simulink model "ur5_simulink_control_2023b"  (R2023b)
settings: Solver=FixedStepAuto  StartTime=0.0  StopTime=inf  FixedStep=0.04  RelTol=1e-3
undefined symbols (not defined in the file or in its folder): data
libraries: robotmaniplib x14, robotcorelib x7, vrlib x2, eeGeneralControl x1
settings Model: Creator=81232  LastModifiedBy=ASUS

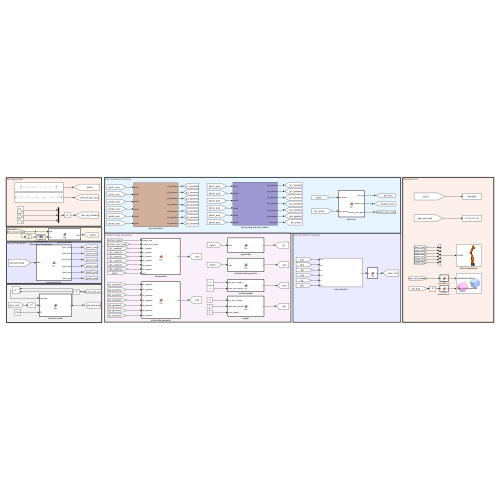
[thumbnail: Simulink's stored preview of the top-level diagram]
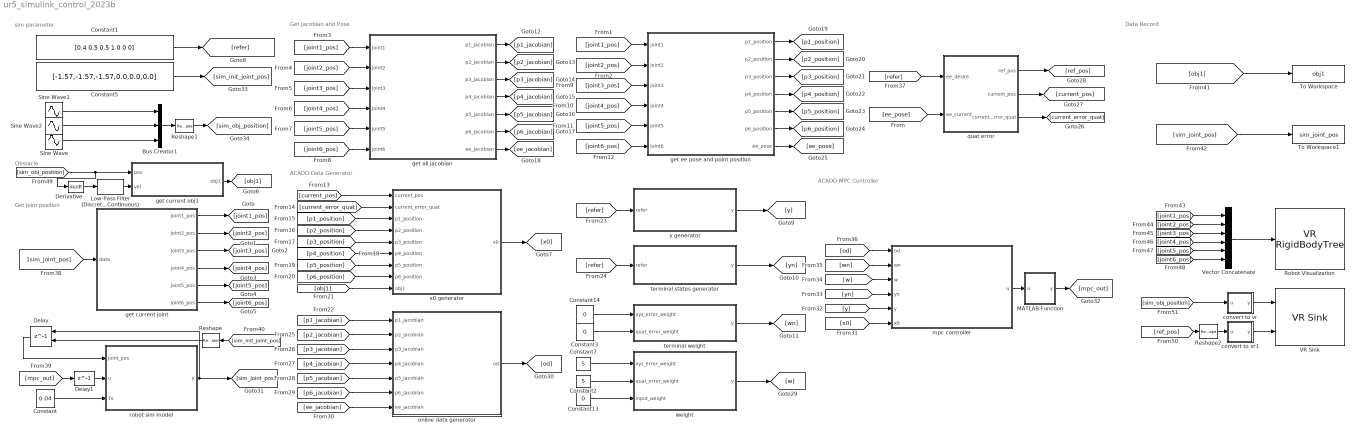
== system ur5_simulink_control_2023b ==
  note: sim parameter
  note: Get joint position
  note: Data Record
  note: Obstacle
  note: ACADO MPC Controller
  note: Get Jacobian and Pose
  note: ACADO Data Generator
  Bus Creator1 : BusCreator  Inputs=3
  Constant : Constant  Value=0.04
  Constant1 : Constant  Value=[0.4 0.5 0.5 1 0 0 0]
  Constant13 : Constant  Value=0
  Constant14 : Constant  Value=0
  Constant2 : Constant  Value=5
  Constant3 : Constant  Value=0
  Constant5 : Constant  Value=[-1.57,-1.57,-1.57,0.0,0.0,0.0]  VectorParams1D=off
  Constant7 : Constant  Value=5
  Delay : Delay  DelayLength=1  InitialConditionSource=Input port  InitialCondition=1
      settings: InputPortMap=u0,p4
  Delay1 : Delay  DelayLength=1
  Derivative : Derivative
  Low-Pass Filter (Discrete or Continuous) : eeGeneralControl/Low-Pass Filter (Discrete or Continuous)  K=1  T=1  B=inf  A=-inf  init_option=Inherited from block input  x0=0  Ts=-1
  MATLAB Function : MATLAB Function  TreatAsAtomicUnit=on
  Reshape : Reshape  OutputDimensionality=Customize  OutputDimensions=[1,6]
  Reshape1 : Reshape  OutputDimensionality=Customize  OutputDimensions=[1,3]
  Reshape2 : Reshape  OutputDimensionality=Customize  OutputDimensions=[1,3]
  Robot Visualization : vrlib/VR RigidBodyTree  VrmlFile=obstacle_robot_scene.x3d  RBT=ur5_model  useRBT=off  Ts=-1  ForceViewerOpen=on
  Sine Wave : Sin  Amplitude=0.3  Bias=0.4  Frequency=0.8  SampleTime=0
  Sine Wave1 : Sin  Amplitude=0.3  Bias=0.4  Frequency=0  SampleTime=0
  Sine Wave2 : Sin  Amplitude=0.3  Bias=0.5  Frequency=0.8  SampleTime=0
  To Workspace : ToWorkspace  VariableName=obj1  SaveFormat=Timeseries  SampleTime=-1
  To Workspace1 : ToWorkspace  VariableName=sim_joint_pos  SaveFormat=Timeseries  SampleTime=-1
  VR Sink : vrlib/VR Sink  InstantiateOnLoad=on  SampleTime=-1  ViewEnable=on  RemoteChange=off  RemoteView=off  FieldsWritten=obstacle.translation.3.1.1.double#refer_point.translation.3.1.1.double  WorldFileName=obstacle_robot_scene.x3d  WorldDescription=Simple Robot Scene  AutoView=off  VideoDimensions=[]  AllowVariableSize=off  FigureProperties=[]
  Vector Concatenate : Concatenate  NumInputs=6
  convert to vr : MATLAB Function  TreatAsAtomicUnit=on
  convert to vr1 : MATLAB Function  TreatAsAtomicUnit=on
  get all jacobian : Subsystem
  get current joint : MATLAB Function  TreatAsAtomicUnit=on
  get current obj1 : MATLAB Function  TreatAsAtomicUnit=on
  get ee pose and point position : Subsystem
  mpc controller : Subsystem
  online data generator : MATLAB Function  TreatAsAtomicUnit=on
  quat error : MATLAB Function  TreatAsAtomicUnit=on
  robot sim model : MATLAB Function  TreatAsAtomicUnit=on
  terminal states generator : MATLAB Function  TreatAsAtomicUnit=on
  terminal weight : MATLAB Function  TreatAsAtomicUnit=on
  weight : MATLAB Function  TreatAsAtomicUnit=on
  x0 generator : MATLAB Function  TreatAsAtomicUnit=on
  y generator : MATLAB Function  TreatAsAtomicUnit=on
  wires:
  get current joint/1(joint1_pos) -> [joint1_pos]
  get current joint/2(joint2_pos) -> [joint2_pos]
  get current joint/3(joint3_pos) -> [joint3_pos]
  get current joint/4(joint4_pos) -> [joint4_pos]
  get current joint/5(joint5_pos) -> [joint5_pos]
  get current joint/6(joint6_pos) -> [joint6_pos]
  [joint1_pos] -> get all jacobian/1(joint1)
  [joint2_pos] -> get all jacobian/2(joint2)
  [joint3_pos] -> get all jacobian/3(joint3)
  [joint4_pos] -> get all jacobian/4(joint4)
  [joint5_pos] -> get all jacobian/5(joint5)
  [joint6_pos] -> get all jacobian/6(joint6)
  get all jacobian/1(p1_jacobian) -> [p1_jacobian]
  get all jacobian/2(p2_jacobian) -> [p2_jacobian]
  get all jacobian/3(p3_jacobian) -> [p3_jacobian]
  get all jacobian/4(p4_jacobian) -> [p4_jacobian]
  get all jacobian/5(p5_jacobian) -> [p5_jacobian]
  get all jacobian/6(p6_jacobian) -> [p6_jacobian]
  get all jacobian/7(ee_jacobian) -> [ee_jacobian]
  [joint6_pos] -> get ee pose and point position/6(joint6)
  [joint4_pos] -> get ee pose and point position/4(joint4)
  [joint1_pos] -> get ee pose and point position/1(joint1)
  [joint2_pos] -> get ee pose and point position/2(joint2)
  [joint5_pos] -> get ee pose and point position/5(joint5)
  [joint3_pos] -> get ee pose and point position/3(joint3)
  [refer] -> quat error/1(ee_desire)
  quat error/3(current_error_quat) -> [current_error_quat]
  get current obj1/1(obj1) -> [obj1]
  get ee pose and point position/1(p1_position) -> [p1_position]
  get ee pose and point position/2(p2_position) -> [p2_position]
  get ee pose and point position/3(p3_position) -> [p3_position]
  get ee pose and point position/4(p4_position) -> [p4_position]
  get ee pose and point position/5(p5_position) -> [p5_position]
  get ee pose and point position/6(p6_position) -> [p6_position]
  get ee pose and point position/7(ee_pose) -> [ee_pose]
  [ee_pose] -> quat error/2(ee_current)
  quat error/2(current_pos) -> [current_pos]
  quat error/1(ref_pos) -> [ref_pos]
  [current_pos] -> x0 generator/1(current_pos)
  [current_error_quat] -> x0 generator/2(current_error_quat)
  [p1_position] -> x0 generator/3(p1_position)
  [p2_position] -> x0 generator/4(p2_position)
  [p3_position] -> x0 generator/5(p3_position)
  [p4_position] -> x0 generator/6(p4_position)
  [p5_position] -> x0 generator/7(p5_position)
  [p6_position] -> x0 generator/8(p6_position)
  [obj1] -> x0 generator/9(obj1)
  x0 generator/1(x0) -> [x0]
  Constant1/1 -> [refer]
  [refer] -> terminal states generator/1(refer)
  terminal states generator/1(y) -> [yn]
  y generator/1(y) -> [y]
  [refer] -> y generator/1(refer)
  terminal weight/1(y) -> [wn]
  Constant7/1 -> weight/1(xyz_error_weight)
  weight/1(y) -> [w]
  Constant14/1 -> terminal weight/1(xyz_error_weight)
  Constant13/1 -> weight/3(input_weight)
  Constant2/1 -> weight/2(quat_error_weight)
  Constant3/1 -> terminal weight/2(quat_error_weight)
  [p1_jacobian] -> online data generator/1(p1_jacobian)
  [p2_jacobian] -> online data generator/2(p2_jacobian)
  [p3_jacobian] -> online data generator/3(p3_jacobian)
  [p4_jacobian] -> online data generator/4(p4_jacobian)
  [p5_jacobian] -> online data generator/5(p5_jacobian)
  [p6_jacobian] -> online data generator/6(p6_jacobian)
  [ee_jacobian] -> online data generator/7(ee_jacobian)
  online data generator/1(od) -> [od]
  [od] -> mpc controller/1(od)
  [wn] -> mpc controller/2(wn)
  [w] -> mpc controller/3(w)
  [yn] -> mpc controller/4(yn)
  [y] -> mpc controller/5(y)
  [x0] -> mpc controller/6(x0)
  Constant/1 -> robot sim model/3(Ts)
  robot sim model/1(y) -> [sim_joint_pos], Delay/1
  Delay/1 -> robot sim model/1(joint_pos)
  [sim_init_joint_pos] -> Reshape/1
  [sim_joint_pos] -> get current joint/1(data)
  Delay1/1 -> robot sim model/2(u)
  Reshape/1 -> Delay/2
  mpc controller/1(u) -> MATLAB Function/1(u)
  MATLAB Function/1(y) -> [mpc_out]
  Constant5/1 -> [sim_init_joint_pos]
  [mpc_out] -> Delay1/1
  [obj1] -> To Workspace/1
  [sim_joint_pos] -> To Workspace1/1
  Vector Concatenate/1 -> Robot Visualization/1
  [joint3_pos] -> Vector Concatenate/3
  [joint1_pos] -> Vector Concatenate/1
  [joint2_pos] -> Vector Concatenate/2
  [joint5_pos] -> Vector Concatenate/5
  [joint6_pos] -> Vector Concatenate/6
  [joint4_pos] -> Vector Concatenate/4
  Reshape1/1 -> [sim_obj_position]
  [sim_obj_position] -> Derivative/1, get current obj1/1(pos)
  [sim_obj_position] -> convert to vr/1(u)
  Sine Wave2/1 -> Bus Creator1/2
  Bus Creator1/1 -> Reshape1/1
  Sine Wave1/1 -> Bus Creator1/1
  Sine Wave/1 -> Bus Creator1/3
  Derivative/1 -> Low-Pass Filter (Discrete or Continuous)/1
  Low-Pass Filter (Discrete or Continuous)/1 -> get current obj1/2(vel)
  convert to vr/1(y) -> VR Sink/1
  convert to vr1/1(y) -> VR Sink/2
  Reshape2/1 -> convert to vr1/1(u)
  [ref_pos] -> Reshape2/1

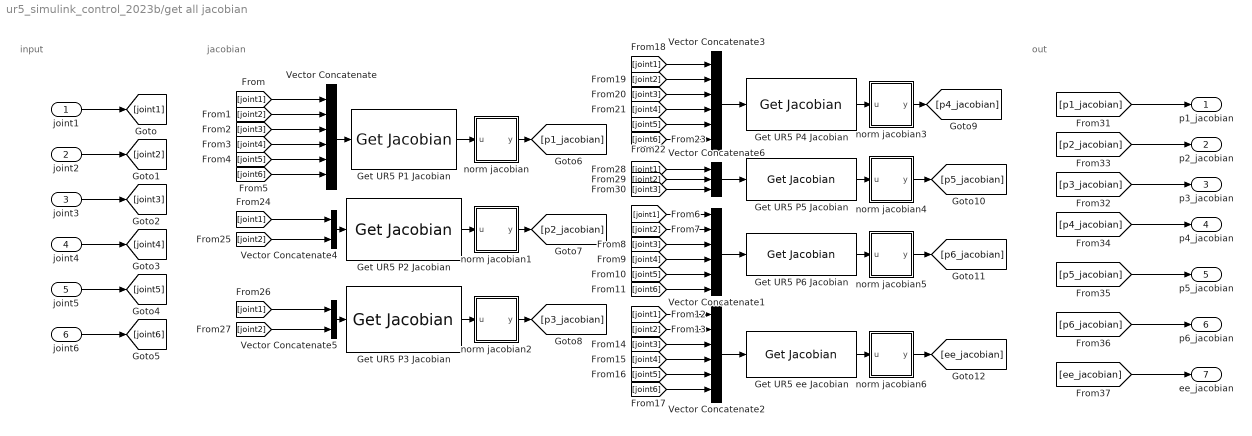
== system ur5_simulink_control_2023b/get all jacobian ==
  note: out
  note: jacobian
  note: input
  joint1 : Inport
  joint2 : Inport  Port=2
  joint3 : Inport  Port=3
  joint4 : Inport  Port=4
  joint5 : Inport  Port=5
  joint6 : Inport  Port=6
  Get UR5 P1 Jacobian : robotmaniplib/Get Jacobian  RigidBodyTree=ur5_model  EndEffector=upper_arm_link  SimulateUsing=Interpreted execution
  Get UR5 P2 Jacobian : robotmaniplib/Get Jacobian  RigidBodyTree=ur5_model_p2  EndEffector=body2  SimulateUsing=Interpreted execution
  Get UR5 P3 Jacobian : robotmaniplib/Get Jacobian  RigidBodyTree=ur5_model_p3  EndEffector=body2  SimulateUsing=Interpreted execution
  Get UR5 P4 Jacobian : robotmaniplib/Get Jacobian  RigidBodyTree=ur5_model  EndEffector=forearm_link  SimulateUsing=Interpreted execution
  Get UR5 P5 Jacobian : robotmaniplib/Get Jacobian  RigidBodyTree=ur5_model_p5  EndEffector=body3  SimulateUsing=Interpreted execution
  Get UR5 P6 Jacobian : robotmaniplib/Get Jacobian  RigidBodyTree=ur5_model  EndEffector=wrist_1_link  SimulateUsing=Interpreted execution
  Get UR5 ee Jacobian : robotmaniplib/Get Jacobian  RigidBodyTree=ur5_model  EndEffector=ee_link  SimulateUsing=Interpreted execution
  Vector Concatenate{,1..3} (4 alike) : Concatenate  NumInputs=6
  Vector Concatenate4 : Concatenate
  Vector Concatenate5 : Concatenate
  Vector Concatenate6 : Concatenate  NumInputs=3
  norm jacobian : MATLAB Function  TreatAsAtomicUnit=on
  norm jacobian1 : MATLAB Function  TreatAsAtomicUnit=on
  norm jacobian2 : MATLAB Function  TreatAsAtomicUnit=on
  norm jacobian3 : MATLAB Function  TreatAsAtomicUnit=on
  norm jacobian4 : MATLAB Function  TreatAsAtomicUnit=on
  norm jacobian5 : MATLAB Function  TreatAsAtomicUnit=on
  norm jacobian6 : MATLAB Function  TreatAsAtomicUnit=on
  p1_jacobian : Outport
  p2_jacobian : Outport  Port=2
  p3_jacobian : Outport  Port=3
  p4_jacobian : Outport  Port=4
  p5_jacobian : Outport  Port=5
  p6_jacobian : Outport  Port=6
  ee_jacobian : Outport  Port=7
  wires:
  joint1/1 -> [joint1]
  joint2/1 -> [joint2]
  joint3/1 -> [joint3]
  joint4/1 -> [joint4]
  joint5/1 -> [joint5]
  joint6/1 -> [joint6]
  Vector Concatenate/1 -> Get UR5 P1 Jacobian/1
  [joint1] -> Vector Concatenate/1
  [joint2] -> Vector Concatenate/2
  [joint3] -> Vector Concatenate/3
  [joint4] -> Vector Concatenate/4
  [joint5] -> Vector Concatenate/5
  [joint6] -> Vector Concatenate/6
  [joint4] -> Vector Concatenate1/4
  [joint3] -> Vector Concatenate1/3
  [joint5] -> Vector Concatenate1/5
  [joint2] -> Vector Concatenate1/2
  [joint1] -> Vector Concatenate1/1
  Vector Concatenate1/1 -> Get UR5 P6 Jacobian/1
  [joint6] -> Vector Concatenate1/6
  [joint4] -> Vector Concatenate3/4
  [joint3] -> Vector Concatenate3/3
  [joint5] -> Vector Concatenate3/5
  [joint2] -> Vector Concatenate3/2
  [joint1] -> Vector Concatenate3/1
  Vector Concatenate3/1 -> Get UR5 P4 Jacobian/1
  [joint6] -> Vector Concatenate3/6
  Vector Concatenate4/1 -> Get UR5 P2 Jacobian/1
  [joint1] -> Vector Concatenate4/1
  [joint2] -> Vector Concatenate4/2
  [joint2] -> Vector Concatenate5/2
  Vector Concatenate5/1 -> Get UR5 P3 Jacobian/1
  [joint1] -> Vector Concatenate5/1
  [joint2] -> Vector Concatenate6/2
  Vector Concatenate6/1 -> Get UR5 P5 Jacobian/1
  [joint1] -> Vector Concatenate6/1
  [joint3] -> Vector Concatenate6/3
  [joint3] -> Vector Concatenate2/3
  [joint2] -> Vector Concatenate2/2
  Vector Concatenate2/1 -> Get UR5 ee Jacobian/1
  [joint5] -> Vector Concatenate2/5
  [joint4] -> Vector Concatenate2/4
  [joint6] -> Vector Concatenate2/6
  [joint1] -> Vector Concatenate2/1
  [p1_jacobian] -> p1_jacobian/1
  [p2_jacobian] -> p2_jacobian/1
  [p3_jacobian] -> p3_jacobian/1
  [p4_jacobian] -> p4_jacobian/1
  [p5_jacobian] -> p5_jacobian/1
  [p6_jacobian] -> p6_jacobian/1
  [ee_jacobian] -> ee_jacobian/1
  Get UR5 P1 Jacobian/1 -> norm jacobian/1(u)
  norm jacobian/1(y) -> [p1_jacobian]
  Get UR5 P2 Jacobian/1 -> norm jacobian1/1(u)
  norm jacobian1/1(y) -> [p2_jacobian]
  norm jacobian2/1(y) -> [p3_jacobian]
  Get UR5 P3 Jacobian/1 -> norm jacobian2/1(u)
  Get UR5 P4 Jacobian/1 -> norm jacobian3/1(u)
  norm jacobian3/1(y) -> [p4_jacobian]
  Get UR5 P5 Jacobian/1 -> norm jacobian4/1(u)
  norm jacobian4/1(y) -> [p5_jacobian]
  Get UR5 P6 Jacobian/1 -> norm jacobian5/1(u)
  norm jacobian5/1(y) -> [p6_jacobian]
  Get UR5 ee Jacobian/1 -> norm jacobian6/1(u)
  norm jacobian6/1(y) -> [ee_jacobian]

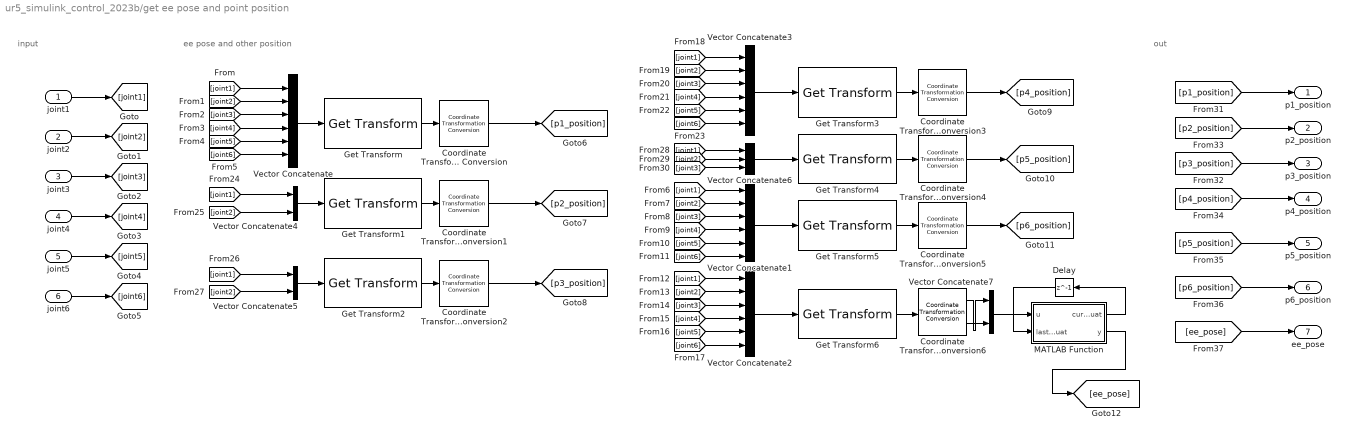
== system ur5_simulink_control_2023b/get ee pose and point position ==
  note: out
  note: ee pose and other position
  note: input
  joint1 : Inport
  joint2 : Inport  Port=2
  joint3 : Inport  Port=3
  joint4 : Inport  Port=4
  joint5 : Inport  Port=5
  joint6 : Inport  Port=6
  Coordinate Transformation Conversion{,1..5} (6 alike) : robotcorelib/Coordinate Transformation Conversion  InputRepresentation=Homogeneous Transformation  InputEulerSequence=ZYX  ShowTrVecInputPort=on  OutputRepresentation=Translation Vector  OutputEulerSequence=ZYX  ShowTrVecOutputPort=on  SimulateUsing=Interpreted execution
  Coordinate Transformation Conversion6 : robotcorelib/Coordinate Transformation Conversion  InputRepresentation=Homogeneous Transformation  InputEulerSequence=ZYX  ShowTrVecInputPort=on  OutputRepresentation=Quaternion  OutputEulerSequence=ZYX  ShowTrVecOutputPort=on  SimulateUsing=Interpreted execution
  Delay : Delay  DelayLength=1  InitialCondition=[0;0;0;0]
  Get Transform : robotmaniplib/Get Transform  RigidBodyTree=ur5_model  SourceBody=upper_arm_link  TargetBody=base_link  SimulateUsing=Interpreted execution
  Get Transform1 : robotmaniplib/Get Transform  RigidBodyTree=ur5_model_p2  SourceBody=body2  TargetBody=base  SimulateUsing=Interpreted execution
  Get Transform2 : robotmaniplib/Get Transform  RigidBodyTree=ur5_model_p3  SourceBody=body2  TargetBody=base  SimulateUsing=Interpreted execution
  Get Transform3 : robotmaniplib/Get Transform  RigidBodyTree=ur5_model  SourceBody=forearm_link  TargetBody=base_link  SimulateUsing=Interpreted execution
  Get Transform4 : robotmaniplib/Get Transform  RigidBodyTree=ur5_model_p5  SourceBody=body3  TargetBody=base  SimulateUsing=Interpreted execution
  Get Transform5 : robotmaniplib/Get Transform  RigidBodyTree=ur5_model  SourceBody=wrist_1_link  TargetBody=base_link  SimulateUsing=Interpreted execution
  Get Transform6 : robotmaniplib/Get Transform  RigidBodyTree=ur5_model  SourceBody=ee_link  TargetBody=base_link  SimulateUsing=Interpreted execution
  MATLAB Function : MATLAB Function  TreatAsAtomicUnit=on
  Vector Concatenate{,1..3} (4 alike) : Concatenate  NumInputs=6
  Vector Concatenate4 : Concatenate
  Vector Concatenate5 : Concatenate
  Vector Concatenate6 : Concatenate  NumInputs=3
  Vector Concatenate7 : Concatenate
  p1_position : Outport
  p2_position : Outport  Port=2
  p3_position : Outport  Port=3
  p4_position : Outport  Port=4
  p5_position : Outport  Port=5
  p6_position : Outport  Port=6
  ee_pose : Outport  Port=7
  wires:
  Get Transform4/1 -> Coordinate Transformation Conversion4/1
  joint1/1 -> [joint1]
  joint2/1 -> [joint2]
  joint3/1 -> [joint3]
  joint4/1 -> [joint4]
  joint5/1 -> [joint5]
  joint6/1 -> [joint6]
  Vector Concatenate/1 -> Get Transform/1
  [joint1] -> Vector Concatenate/1
  [joint2] -> Vector Concatenate/2
  [joint3] -> Vector Concatenate/3
  [joint4] -> Vector Concatenate/4
  [joint5] -> Vector Concatenate/5
  [joint6] -> Vector Concatenate/6
  [joint4] -> Vector Concatenate1/4
  [joint3] -> Vector Concatenate1/3
  [joint5] -> Vector Concatenate1/5
  [joint2] -> Vector Concatenate1/2
  [joint1] -> Vector Concatenate1/1
  Vector Concatenate1/1 -> Get Transform5/1
  [joint6] -> Vector Concatenate1/6
  [joint4] -> Vector Concatenate3/4
  [joint3] -> Vector Concatenate3/3
  [joint5] -> Vector Concatenate3/5
  [joint2] -> Vector Concatenate3/2
  [joint1] -> Vector Concatenate3/1
  Vector Concatenate3/1 -> Get Transform3/1
  [joint6] -> Vector Concatenate3/6
  Vector Concatenate4/1 -> Get Transform1/1
  [joint1] -> Vector Concatenate4/1
  [joint2] -> Vector Concatenate4/2
  [joint2] -> Vector Concatenate5/2
  Vector Concatenate5/1 -> Get Transform2/1
  [joint1] -> Vector Concatenate5/1
  [joint2] -> Vector Concatenate6/2
  Vector Concatenate6/1 -> Get Transform4/1
  [joint1] -> Vector Concatenate6/1
  [joint3] -> Vector Concatenate6/3
  [joint3] -> Vector Concatenate2/3
  [joint2] -> Vector Concatenate2/2
  Vector Concatenate2/1 -> Get Transform6/1
  [joint5] -> Vector Concatenate2/5
  [joint4] -> Vector Concatenate2/4
  [joint6] -> Vector Concatenate2/6
  [joint1] -> Vector Concatenate2/1
  [p1_position] -> p1_position/1
  [p2_position] -> p2_position/1
  [p3_position] -> p3_position/1
  [p4_position] -> p4_position/1
  [p5_position] -> p5_position/1
  [p6_position] -> p6_position/1
  [ee_pose] -> ee_pose/1
  Get Transform/1 -> Coordinate Transformation Conversion/1
  Coordinate Transformation Conversion/1 -> [p1_position]
  Coordinate Transformation Conversion1/1 -> [p2_position]
  Get Transform1/1 -> Coordinate Transformation Conversion1/1
  Get Transform2/1 -> Coordinate Transformation Conversion2/1
  Coordinate Transformation Conversion2/1 -> [p3_position]
  Get Transform3/1 -> Coordinate Transformation Conversion3/1
  Coordinate Transformation Conversion3/1 -> [p4_position]
  Coordinate Transformation Conversion4/1 -> [p5_position]
  Get Transform5/1 -> Coordinate Transformation Conversion5/1
  Coordinate Transformation Conversion5/1 -> [p6_position]
  Get Transform6/1 -> Coordinate Transformation Conversion6/1
  Coordinate Transformation Conversion6/2 -> Vector Concatenate7/1
  Coordinate Transformation Conversion6/1 -> Vector Concatenate7/2
  Vector Concatenate7/1 -> MATLAB Function/1(u)
  MATLAB Function/1(current_quat) -> Delay/1
  MATLAB Function/2(y) -> [ee_pose]
  Delay/1 -> MATLAB Function/2(last_quat)

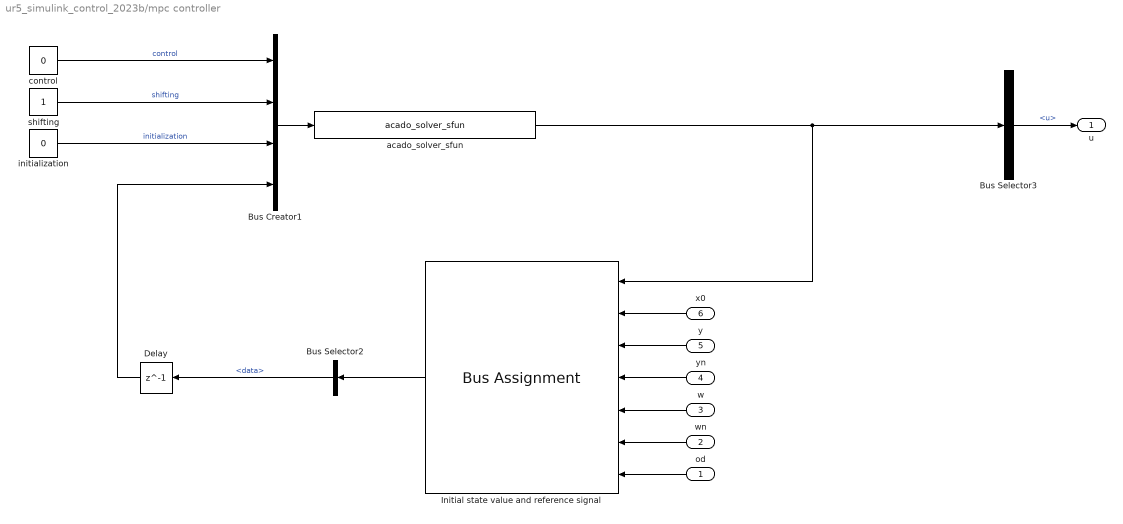
== system ur5_simulink_control_2023b/mpc controller ==
  od : Inport
  wn : Inport  Port=2
  w : Inport  Port=3
  yn : Inport  Port=4
  y : Inport  Port=5
  x0 : Inport  Port=6
  Bus Creator1 : BusCreator  Inputs=4  OutDataTypeStr=Bus: ACADOinput
  Bus Selector2 : BusSelector  OutputSignals=data
  Bus Selector3 : BusSelector  OutputSignals=data.u
  Delay : Delay  DelayLength=1
  Initial state value and reference signal : BusAssignment  AssignedSignals=data.x0,data.y,data.yN,data.W,data.WN,data.od
  acado_solver_sfun : S-Function  FunctionName=acado_solver_sfun  SFunctionDeploymentMode=off  EnableBusSupport=off  mask(Legacy Function){SFunctionSpec=acado_step(ACADOinput u1[1], ACADOoutput y1[1]), ShowSpec=on}
      mask prompts: ShowSpec "显示函数设定"
      mask help:
      | 此模块允许您调用由以下代码继承工具定义指定的已有函数:
      | def.SFunctionName = 'acado_solver_sfun';
      | def.OutputFcnSpec = 'acado_step(ACADOinput u1[1], ACADOoutput y1[1])';
      | def.StartFcnSpec = 'acado_initialize( void )';
      | def.TerminateFcnSpec = 'acado_cleanup( void )';
      | def.HeaderFiles = {'acado_common.h', 'acado_solver_sfunction.h'};
      | def.SourceFiles = {'acado_solver.c', 'acado_integrator.c', 'acado_auxiliary_functions.c', 'acado_solver_sfunction.c', 'acado_qpoases3_interface.c', 'qpoases3\src\Bounds.c', 'qpoases3\src\Constraints.c', 'qpoases3\src\Indexlist.c', 'qpoases3\src\Matrices.c', 'qpoases3\src\MessageHandling.c', 'qpoases3\src\Options.c', 'qpoases3\src\Flipper.c', 'qpoases3\src\QProblem.c', 'qpoases3\src\QProblemB.c', 'qpoases3\src\Utils.c'};
      mask Help: <p>此模块是由代码继承工具自动生成的。有关此工具的详细帮助，请调用<a href="matlab:legacy_code('help')"> legacy_code('help')</a>.</p>
      mask Callback ShowSpec:
      | if strcmp(get_param(gcbh, 'ShowSpec'), 'on')
      |   set_param(gcbh, 'MaskDisplay', sprintf('fprintf(''%s'');', get_param(gcbh, 'SFunctionSpec')));
      | else
      |   set_param(gcbh, 'MaskDisplay', sprintf('fprintf(''%s'');', get_param(gcbh, 'FunctionName')));
      | end
      mask Display: fprintf('acado_step(ACADOinput u1[1], ACADOoutput y1[1])');
  control : Constant  Value=0  OutDataTypeStr=int32
  initialization : Constant  Value=0  OutDataTypeStr=int32
  shifting : Constant  OutDataTypeStr=int32
  u : Outport
  wires:
  Bus Creator1/1 -> acado_solver_sfun/1
  acado_solver_sfun/1 -> Initial state value and reference signal/1, Bus Selector3/1
  Initial state value and reference signal/1 -> Bus Selector2/1
  initialization/1 -> Bus Creator1/3  "initialization"
  shifting/1 -> Bus Creator1/2  "shifting"
  control/1 -> Bus Creator1/1  "control"
  w/1 -> Initial state value and reference signal/5
  Bus Selector2/1 -> Delay/1  "<data>"
  wn/1 -> Initial state value and reference signal/6
  Delay/1 -> Bus Creator1/4
  od/1 -> Initial state value and reference signal/7
  yn/1 -> Initial state value and reference signal/4
  y/1 -> Initial state value and reference signal/3
  x0/1 -> Initial state value and reference signal/2
  Bus Selector3/1 -> u/1  "<u>"

== matlab function ur5_simulink_control_2023b/get current obj1 ==
  data: obj1 output; pos input; vel input
function obj1  = fcn(pos, vel)
obj1_px = pos(1);
obj1_py = pos(2);
obj1_pz = pos(3);
obj1_vx = vel(1);
obj1_vy = vel(2);
obj1_vz = vel(3);
obj1 = [obj1_px,obj1_py,obj1_pz,obj1_vx,obj1_vy,obj1_vz];

== matlab function ur5_simulink_control_2023b/terminal states generator ==
  data: refer input; y output
function y = fcn(refer)
y = zeros(1,30);
y(1,1)= refer(1);
y(1,2)= refer(2);
y(1,3)= refer(3);

== matlab function ur5_simulink_control_2023b/online data generator ==
  data: p1_jacobian input; od output; p2_jacobian input; p3_jacobian input; p4_jacobian input; p5_jacobian input; p6_jacobian input; ee_jacobian input
function od = fcn(p1_jacobian,p2_jacobian,p3_jacobian,p4_jacobian,p5_jacobian,p6_jacobian,ee_jacobian)
od = zeros(1,270);
od(1:6) =  reshape(p1_jacobian(1:3,1:2)',[1,6]);
od(7:12) =  reshape(p2_jacobian(1:3,1:2)',[1,6]);
od(13:18) =  reshape(p3_jacobian(1:3,1:2)',[1,6]);
od(19:27) =  reshape(p4_jacobian(1:3,1:3)',[1,9]);
od(28:36) =  reshape(p5_jacobian(1:3,1:3)',[1,9]);
od(37:54) =  reshape(p6_jacobian(1:3,1:6)',[1,18]);
od(55:90) =  reshape(ee_jacobian(1:6,1:6)',[1,36]);
od(91:180) = od(1:90);
od(181:270) = od(1:90);

== matlab function ur5_simulink_control_2023b/y generator ==
  data: refer input; y output
function y = fcn(refer)
y = zeros(1,72);
for i = 1:2
    y(1,(i-1)*36+1)= refer(1);
    y(1,(i-1)*36+2)= refer(2);
    y(1,(i-1)*36+3)= refer(3);
end

== matlab function ur5_simulink_control_2023b/weight ==
  data: xyz_error_weight input; quat_error_weight input; y output; input_weight input
function y = fcn(xyz_error_weight, quat_error_weight, input_weight)
a =zeros(36,36);
a(1:3,1:3) = xyz_error_weight*eye(3);
a(4:6,4:6) = quat_error_weight*eye(3);
a(31:36,31:36) = input_weight*eye(6);
y =zeros(1,1296);
for i = 1:36
    y(1,(i-1)*36+1:(i-1)*36+36) = a(i,1:36);
end

== matlab function ur5_simulink_control_2023b/robot sim model ==
  data: joint_pos input size=[1,6]; u input size=[1,6]; y output size=[1,6]; Ts input
function y = fcn(joint_pos,u,Ts)
a = u;

y = joint_pos + Ts*a(1:6);

== matlab function ur5_simulink_control_2023b/get all jacobian/norm jacobian ==
  data: u input; y output
function y = fcn(u)
lastThreeColumns = u(4:6, :);
y = lastThreeColumns;

== matlab function ur5_simulink_control_2023b/terminal weight ==
  data: xyz_error_weight input; y output; quat_error_weight input
function y = fcn(xyz_error_weight, quat_error_weight)
a =zeros(30,30);
a(1:3,1:3) = xyz_error_weight*eye(3);
a(4:6,4:6) = quat_error_weight*eye(3);
y =zeros(1,900);
for i = 1:30
    y(1,(i-1)*30+1:(i-1)*30+30) = a(i,1:30);
end

== matlab function ur5_simulink_control_2023b/MATLAB Function ==
  data: u input; y output
function y = fcn(u)

y = u(1:6);

== matlab function ur5_simulink_control_2023b/convert to vr ==
  data: u input; y output
function y = fcn(u)
y = u;
y(1)= u(1);
y(2)= u(3);
y(3)= -u(2);

== matlab function ur5_simulink_control_2023b/convert to vr1 ==
  data: u input; y output
function y = fcn(u)
y = u;
y(1)= u(1);
y(2)= u(3);
y(3)= -u(2);

== matlab function ur5_simulink_control_2023b/get ee pose and point position/MATLAB Function ==
  data: current_quat output; u input; y output; last_quat input size=[4,1]
function [current_quat,y] = fcn(u, last_quat)
current_quat = u(4:7);
quat_dot = current_quat(1)*last_quat(1)+current_quat(2)*last_quat(2)+current_quat(3)*last_quat(3)++current_quat(4)*last_quat(4);
if(quat_dot<0)
    current_quat = -1*current_quat;
end
y = [u(1:3);current_quat];

== matlab function ur5_simulink_control_2023b/get current joint ==
  data: joint1_pos output; joint2_pos output; joint3_pos output; joint4_pos output; joint5_pos output; joint6_pos output; data input
function [joint1_pos,joint2_pos,joint3_pos,joint4_pos,joint5_pos,joint6_pos] = fcn(data)
joint1_pos = data(1);
joint2_pos = data(2);
joint3_pos = data(3);
joint4_pos = data(4);
joint5_pos = data(5);
joint6_pos = data(6);

== matlab function ur5_simulink_control_2023b/get all jacobian/norm jacobian1 ==
  data: u input; y output
function y = fcn(u)
lastThreeColumns = u(4:6, :);
y = lastThreeColumns;

== matlab function ur5_simulink_control_2023b/get all jacobian/norm jacobian2 ==
  data: u input; y output
function y = fcn(u)
lastThreeColumns = u(4:6, :);
y = lastThreeColumns;

== matlab function ur5_simulink_control_2023b/get all jacobian/norm jacobian3 ==
  data: u input; y output
function y = fcn(u)
lastThreeColumns = u(4:6, :);
y = lastThreeColumns;

== matlab function ur5_simulink_control_2023b/get all jacobian/norm jacobian4 ==
  data: u input; y output
function y = fcn(u)
lastThreeColumns = u(4:6, :);
y = lastThreeColumns;

== matlab function ur5_simulink_control_2023b/get all jacobian/norm jacobian5 ==
  data: u input; y output
function y = fcn(u)
lastThreeColumns = u(4:6, :);
y = lastThreeColumns;

== matlab function ur5_simulink_control_2023b/get all jacobian/norm jacobian6 ==
  data: u input; y output
function y = fcn(u)
firstThreeColumns =u(1:3, :);
lastThreeColumns = u(4:6, :);
y = [lastThreeColumns;firstThreeColumns];

== matlab function ur5_simulink_control_2023b/x0 generator ==
  data: current_pos input; x0 output; current_error_quat input; p1_position input; p2_position input; p3_position input; p4_position input; p5_position input; p6_position input; obj1 input
function x0 = fcn(current_pos, current_error_quat, p1_position, p2_position, p3_position, p4_position, p5_position, p6_position, obj1)

x0 = zeros(1,30);
x0(1:3) = current_pos(1:3);
x0(4:6) = -current_error_quat;
x0(7:9)= p1_position;
x0(10:12)= p2_position;
x0(13:15)= p3_position;
x0(16:18)= p4_position;
x0(19:21)= p5_position;
x0(22:24)= p6_position;
x0(25:30)= obj1;

== matlab function ur5_simulink_control_2023b/quat error ==
  data: ee_desire input; ref_pos output; ee_current input; current_pos output; current_error_quat output
function [ref_pos,current_pos,current_error_quat] = fcn(ee_desire,ee_current)
current_pos = ee_current(1:3);
ref_pos = ee_desire(1:3);
current_quat = ee_current(4:7);
ref_quat = ee_desire(4:7);
sym_ref = [0,-ref_quat(4),ref_quat(3);ref_quat(4),0,-ref_quat(2);-ref_quat(3),ref_quat(2),0];
current_error_quat =current_quat(1)*ref_quat(2:4)-ref_quat(1)*current_quat(2:4)-sym_ref*current_quat(2:4);
